simulink model "IPC4M"  (R2015a)
settings: Solver=ode3  SolverMode=SingleTasking  StartTime=0.0  StopTime=30.0  FixedStep=1e-2  RelTol=1e-7
values from neighbouring files (symbols this model uses):
  d = 5    [IPC4Minit.m]
  delta = 5    [IPC4Minit.m]
  g = [0;0;-9.81]    [IPC4Minit.m]
  j0 = 10    [IPC4Minit.m]
  j1 = 10    [IPC4Minit.m]
  j2 = 10    [IPC4Minit.m]
  j3 = 10    [IPC4Minit.m]
  j4 = 10    [IPC4Minit.m]
  k = 10    [IPC4Minit.m]
  kappa = 10    [IPC4Minit.m]
  Kc = 10    [IPC4Minit.m]
  l = [1 1 1 1]    [IPC4Minit.m]
  m0 = 10    [IPC4Minit.m]
  m1 = 10    [IPC4Minit.m]
  m2 = 10    [IPC4Minit.m]
  m3 = 10    [IPC4Minit.m]
  m4 = 10    [IPC4Minit.m]
libraries: aerolibutil x4, dspinverses x3, simulink x1
settings Model: CovSFcnEnable=off  Creator=Martin  LastModifiedBy=mangerer
settings SolverCC: ZeroCrossAlgorithm=Adaptive
settings DataIOCC: LimitDataPoints=off
settings OptimizationCC: BlockReduction=off  BooleanDataType=off
settings DebuggingCC: SaveWithParameterizedLinksMsg=none  UnderspecifiedInitializationDetection=Classic  MergeDetectMultiDrivingBlocksExec=none  SignalResolutionControl=TryResolveAllWithWarning
settings HardwareCC: TargetBitPerLong=64  TargetBitPerPointer=64  TargetLongLongMode=on  TargetIntDivRoundTo=Zero  TargetEndianess=LittleEndian  TargetWordSize=64  TargetHWDeviceType=MATLAB Host  ProdEqTarget=off

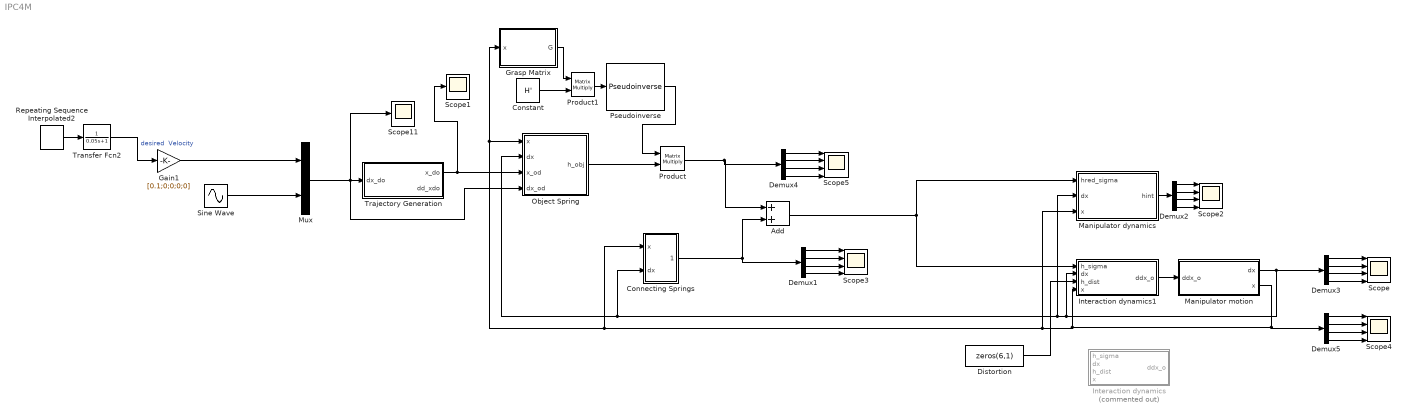
== system IPC4M ==
  Add : Sum
  Connecting Springs : Subsystem
  Constant : Constant  Value=H'
  Demux{1..5} (5 alike) : Demux
  Distortion : Constant  Value=zeros(6,1)
  Gain1 : Gain  Gain=[0.1;0;0;0;0]
  Grasp Matrix : MATLAB Function  TreatAsAtomicUnit=on
  Interaction dynamics : Subsystem  Commented=on
  Interaction dynamics1 : Subsystem
  Manipulator dynamics : Subsystem
  Manipulator motion : Subsystem
  Mux : Mux  Inputs=2
  Object Spring : Subsystem
  Product : Product  Multiplication=Matrix(*)
  Product1 : Product  Multiplication=Matrix(*)
  Pseudoinverse : dspinverses/Pseudoinverse  wanterr=off
  Repeating Sequence Interpolated2 : simulink/Sources/Repeating Sequence Interpolated  OutValues=[0 0 1 1 0 0].'  TimeValues=[0 0.1 1.5 2 2.5 3].'  LookUpMeth=Interpolation-Use End Values  tsamp=0.01  OutMin=[]  OutMax=[]  OutDataTypeStr=double  OutputDataTypeScalingMode=double  OutDataType=fixdt(0,8)  OutScaling=2^-10
  Scope{,2..5} (5 alike) : Scope  NumInputPorts=4
      Scope settings: ShowLegends=on  TimeRange=3  YMin=-15~-12.5~-12.5~-15  YMax=15~15~15~15
      Scope2 settings: ShowLegends=on  TimeRange=10  YMin=-150~-150~-150~-150  YMax=150~150~150~150  SaveName=ScopeData2
      Scope3 settings: ShowLegends=on  TimeRange=3  YMin=-15~-12.5~-12.5~-15  YMax=15~15~15~15  SaveName=ScopeData13
      Scope4 settings: ShowLegends=on  YMin=-5~-5~-5~-5  YMax=5~5~5~5  SaveName=ScopeData10
      Scope5 settings: ShowLegends=on  TimeRange=3  YMin=-15~-12.5~-12.5~-15  YMax=15~15~15~15  SaveName=ScopeData16
  Scope1 : Scope
      settings: YMin=0  YMax=0.9
  Scope11 : Scope
      settings: YMin=0.9984  YMax=1  SaveName=ScopeData26
  Sine Wave : Sin  Amplitude=0  Frequency=1*pi  SampleTime=0
  Trajectory Generation : Subsystem
  Transfer Fcn2 : TransferFcn  Denominator=[0.05 1]
  wires:
  Manipulator dynamics/1(hint) -> Demux2/1
  Demux2/1 -> Scope2/1
  Demux2/2 -> Scope2/2
  Demux2/4 -> Scope2/4
  Demux3/1 -> Scope/1
  Demux3/2 -> Scope/2
  Demux3/3 -> Scope/3
  Demux3/4 -> Scope/4
  Demux5/1 -> Scope4/1
  Demux5/2 -> Scope4/2
  Demux5/3 -> Scope4/3
  Demux5/4 -> Scope4/4
  Gain1/1 -> Mux/1
  Manipulator motion/1(dx) -> Demux3/1, Connecting Springs/2(dx), Object Spring/2(dx), Manipulator dynamics/2(dx), Interaction dynamics1/2(dx)
  Mux/1 -> Scope11/1, Object Spring/4(dx_od), Trajectory Generation/1(dx_do)
  Manipulator motion/2(x) -> Demux5/1, Grasp Matrix/1(x), Object Spring/1(x), Connecting Springs/1(x), Manipulator dynamics/3(x), Interaction dynamics1/4(x)
  Sine Wave/1 -> Mux/2
  Demux2/3 -> Scope2/3
  Interaction dynamics1/1(ddx_o) -> Manipulator motion/1(ddx_o)
  Distortion/1 -> Interaction dynamics1/3(h_dist)
  Trajectory Generation/1(x_do) -> Scope1/1, Object Spring/3(x_od)
  Object Spring/1(h_obj) -> Product/2
  Add/1 -> Manipulator dynamics/1(hred_sigma), Interaction dynamics1/1(h_sigma)
  Repeating Sequence Interpolated2/1 -> Transfer Fcn2/1
  Transfer Fcn2/1 -> Gain1/1  "desired  Velocity"
  Demux1/1 -> Scope3/1
  Demux1/2 -> Scope3/2
  Demux1/3 -> Scope3/3
  Demux1/4 -> Scope3/4
  Connecting Springs/1(h_con) -> Add/2, Demux1/1
  Demux4/1 -> Scope5/1
  Demux4/2 -> Scope5/2
  Demux4/3 -> Scope5/3
  Demux4/4 -> Scope5/4
  Product/1 -> Demux4/1, Add/1
  Grasp Matrix/1(G) -> Product1/1
  Constant/1 -> Product1/2
  Product1/1 -> Pseudoinverse/1
  Pseudoinverse/1 -> Product/1

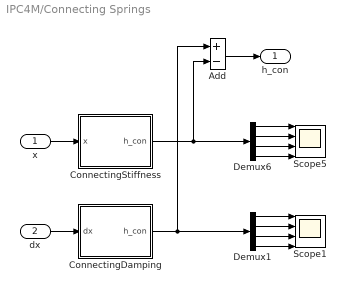
== system IPC4M/Connecting Springs ==
  x : Inport
  dx : Inport  Port=2
  Add : Sum  Inputs=+-
  ConnectingDamping : MATLAB Function  TreatAsAtomicUnit=on
  ConnectingStiffness : MATLAB Function  TreatAsAtomicUnit=on
  Demux1 : Demux
  Demux6 : Demux
  Scope1 : Scope  NumInputPorts=4
      settings: ShowLegends=on  YMin=-10~-50~-80~-80  YMax=80~80~10~50  SaveName=ScopeData12
  Scope5 : Scope  NumInputPorts=4
      settings: ShowLegends=on  YMin=-10~-50~-80~-80  YMax=80~80~10~50  SaveName=ScopeData11
  h_con : Outport
  wires:
  Demux6/1 -> Scope5/1
  Demux6/2 -> Scope5/2
  Demux6/3 -> Scope5/3
  Demux6/4 -> Scope5/4
  ConnectingStiffness/1(h_con) -> Add/2, Demux6/1
  Demux1/1 -> Scope1/1
  Demux1/2 -> Scope1/2
  Demux1/3 -> Scope1/3
  Demux1/4 -> Scope1/4
  ConnectingDamping/1(h_con) -> Add/1, Demux1/1
  x/1 -> ConnectingStiffness/1(x)
  dx/1 -> ConnectingDamping/1(dx)
  Add/1 -> h_con/1

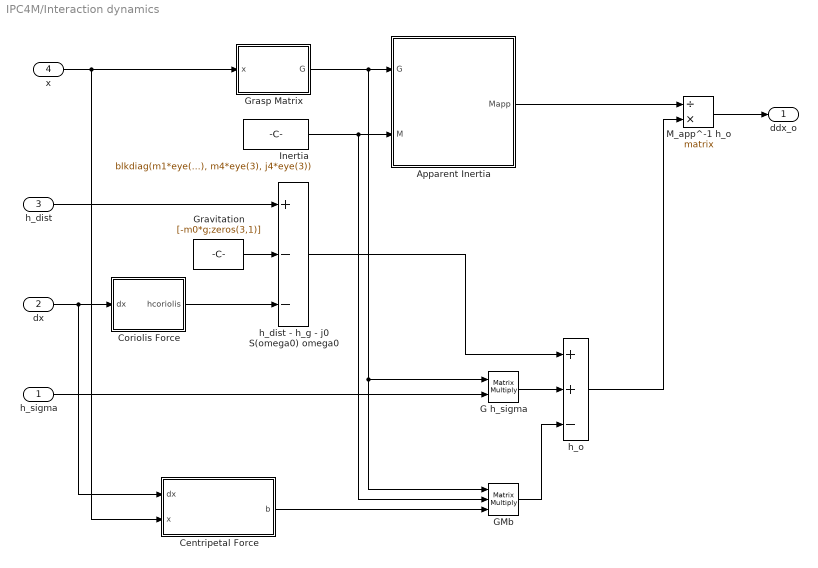
== system IPC4M/Interaction dynamics ==
  h_sigma : Inport
  dx : Inport  Port=2
  h_dist : Inport  Port=3
  x : Inport  Port=4
  Apparent Inertia : MATLAB Function  TreatAsAtomicUnit=on
  Centripetal Force : MATLAB Function  TreatAsAtomicUnit=on
  Coriolis Force : MATLAB Function  TreatAsAtomicUnit=on
  G h_sigma : Product  Multiplication=Matrix(*)
  GMb : Product  Inputs=***  Multiplication=Matrix(*)
  Grasp Matrix : MATLAB Function  TreatAsAtomicUnit=on
  Gravitation : Constant  Value=[-m0*g;zeros(3,1)]
  Inertia : Constant  Value=blkdiag(m1*eye(3), j1*eye(3), m2*eye(3), j2*eye(3), m3*eye(3), j3*eye(3), m4*eye(3), j4*eye(3))
  M_app^-1 h_o : Product  Inputs=/*  Multiplication=Matrix(*)
  "h_dist - h_g - j0 S(omega0) omega0 " : Sum  Inputs=+--
  h_o : Sum  Inputs=++-
  ddx_o : Outport
  wires:
  Grasp Matrix/1(G) -> G h_sigma/1, GMb/1, Apparent Inertia/1(G)
  Inertia/1 -> GMb/2, Apparent Inertia/2(M)
  Apparent Inertia/1(Mapp) -> M_app^-1 h_o/1
  h_o/1 -> M_app^-1 h_o/2
  G h_sigma/1 -> h_o/2
  h_sigma/1 -> G h_sigma/2
  "h_dist - h_g - j0 S(omega0) omega0 "/1 -> h_o/1
  h_dist/1 -> "h_dist - h_g - j0 S(omega0) omega0 "/1
  Gravitation/1 -> "h_dist - h_g - j0 S(omega0) omega0 "/2
  dx/1 -> Centripetal Force/1(dx), Coriolis Force/1(dx)
  Coriolis Force/1(hcoriolis) -> "h_dist - h_g - j0 S(omega0) omega0 "/3
  GMb/1 -> h_o/3
  Centripetal Force/1(b) -> GMb/3
  M_app^-1 h_o/1 -> ddx_o/1
  x/1 -> Centripetal Force/2(x), Grasp Matrix/1(x)

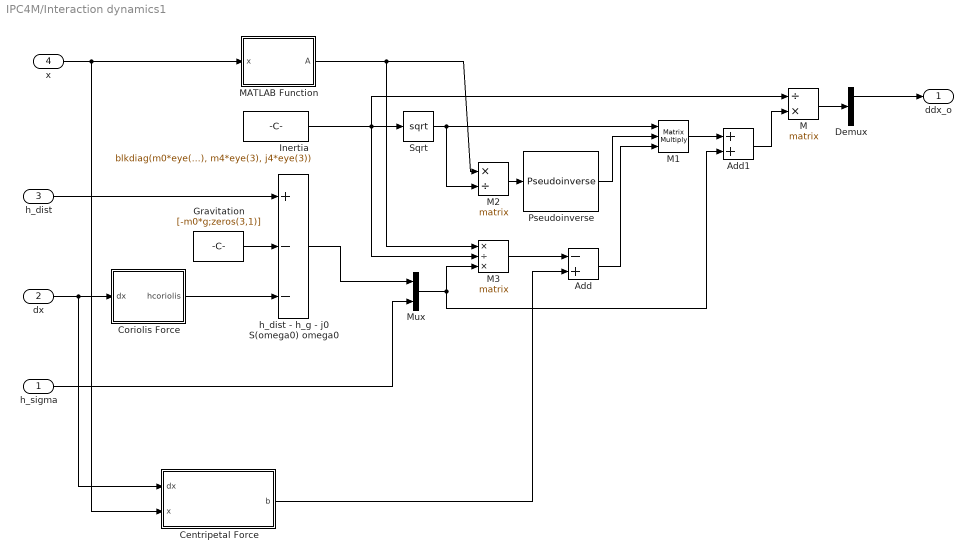
== system IPC4M/Interaction dynamics1 ==
  h_sigma : Inport
  dx : Inport  Port=2
  h_dist : Inport  Port=3
  x : Inport  Port=4
  Add : Sum  Inputs=-+
  Add1 : Sum
  Centripetal Force : MATLAB Function  TreatAsAtomicUnit=on
  Coriolis Force : MATLAB Function  TreatAsAtomicUnit=on
  Demux : Demux  Outputs=5
  Gravitation : Constant  Value=[-m0*g;zeros(3,1)]
  Inertia : Constant  Value=blkdiag(m0*eye(3),j0*eye(3),m1*eye(3), j1*eye(3), m2*eye(3), j2*eye(3), m3*eye(3), j3*eye(3), m4*eye(3), j4*eye(3))
  M : Product  Inputs=/*  Multiplication=Matrix(*)
  M1 : Product  Inputs=***  Multiplication=Matrix(*)
  M2 : Product  Inputs=*/  Multiplication=Matrix(*)
  M3 : Product  Inputs=*/*  Multiplication=Matrix(*)
  MATLAB Function : MATLAB Function  TreatAsAtomicUnit=on
  Mux : Mux  Inputs=2
  Pseudoinverse : dspinverses/Pseudoinverse  wanterr=off
  Sqrt : Sqrt  SaturateOnIntegerOverflow=on
  "h_dist - h_g - j0 S(omega0) omega0 " : Sum  Inputs=+--
  ddx_o : Outport
  wires:
  h_dist/1 -> "h_dist - h_g - j0 S(omega0) omega0 "/1
  Gravitation/1 -> "h_dist - h_g - j0 S(omega0) omega0 "/2
  dx/1 -> Centripetal Force/1(dx), Coriolis Force/1(dx)
  Coriolis Force/1(hcoriolis) -> "h_dist - h_g - j0 S(omega0) omega0 "/3
  x/1 -> MATLAB Function/1(x), Centripetal Force/2(x)
  Inertia/1 -> M/1, M3/2, Sqrt/1
  Sqrt/1 -> M2/2, M1/1
  MATLAB Function/1(A) -> M3/1, M2/1
  M2/1 -> Pseudoinverse/1
  Pseudoinverse/1 -> M1/2
  Add/1 -> M1/3
  Centripetal Force/1(b) -> Add/2
  M3/1 -> Add/1
  Mux/1 -> Add1/2, M3/3
  "h_dist - h_g - j0 S(omega0) omega0 "/1 -> Mux/1
  h_sigma/1 -> Mux/2
  M/1 -> Demux/1
  Demux/1 -> ddx_o/1
  M1/1 -> Add1/1
  Add1/1 -> M/2

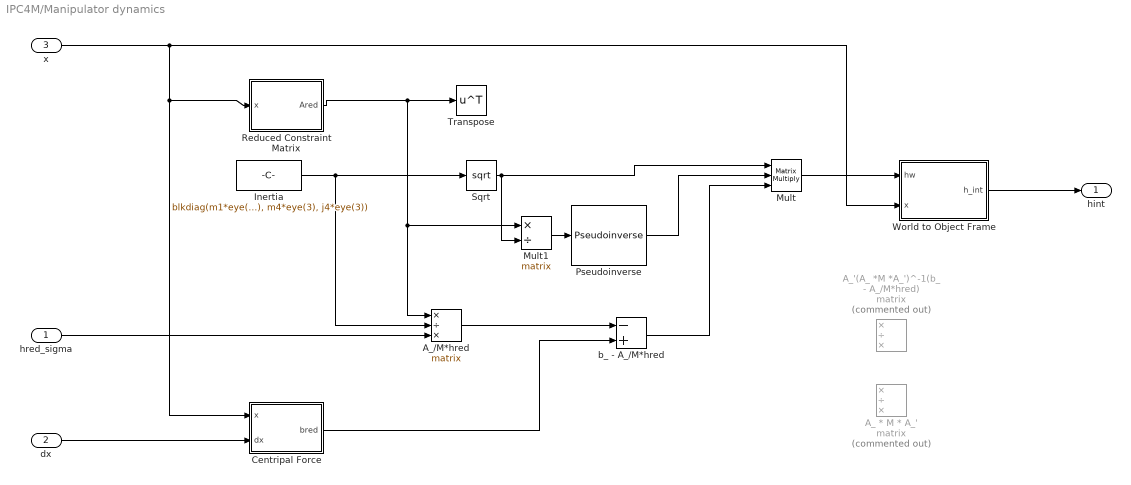
== system IPC4M/Manipulator dynamics ==
  hred_sigma : Inport
  dx : Inport  Port=2
  x : Inport  Port=3
  A_ * M * A_' : Product  Commented=on  Inputs=*/*  Multiplication=Matrix(*)
  A_'(A_ *M *A_')^-1(b_ - A_/M*hred) : Product  Commented=on  Inputs=*/*  Multiplication=Matrix(*)
  A_/M*hred : Product  Inputs=*/*  Multiplication=Matrix(*)
  Centripal Force : MATLAB Function  TreatAsAtomicUnit=on
  Inertia : Constant  Value=blkdiag(m1*eye(3), j1*eye(3), m2*eye(3), j2*eye(3), m3*eye(3), j3*eye(3), m4*eye(3), j4*eye(3))
  Mult : Product  Inputs=***  Multiplication=Matrix(*)
  Mult1 : Product  Inputs=*/  Multiplication=Matrix(*)
  Pseudoinverse : dspinverses/Pseudoinverse  wanterr=off
  Reduced Constraint Matrix : MATLAB Function  TreatAsAtomicUnit=on
  Sqrt : Sqrt  SaturateOnIntegerOverflow=on
  Transpose : Math  Operator=transpose  SaturateOnIntegerOverflow=on
  World to Object Frame : MATLAB Function  TreatAsAtomicUnit=on
  b_ - A_/M*hred : Sum  Inputs=-+
  hint : Outport
  wires:
  Reduced Constraint Matrix/1(Ared) -> Transpose/1, A_/M*hred/1, Mult1/1
  Inertia/1 -> Sqrt/1, A_/M*hred/2
  dx/1 -> Centripal Force/2(dx)
  A_/M*hred/1 -> b_ - A_/M*hred/1
  hred_sigma/1 -> A_/M*hred/3
  World to Object Frame/1(h_int) -> hint/1
  x/1 -> Centripal Force/1(x), Reduced Constraint Matrix/1(x), World to Object Frame/2(x)
  Centripal Force/1(bred) -> b_ - A_/M*hred/2
  Mult/1 -> World to Object Frame/1(hw)
  b_ - A_/M*hred/1 -> Mult/3
  Sqrt/1 -> Mult1/2, Mult/1
  Mult1/1 -> Pseudoinverse/1
  Pseudoinverse/1 -> Mult/2

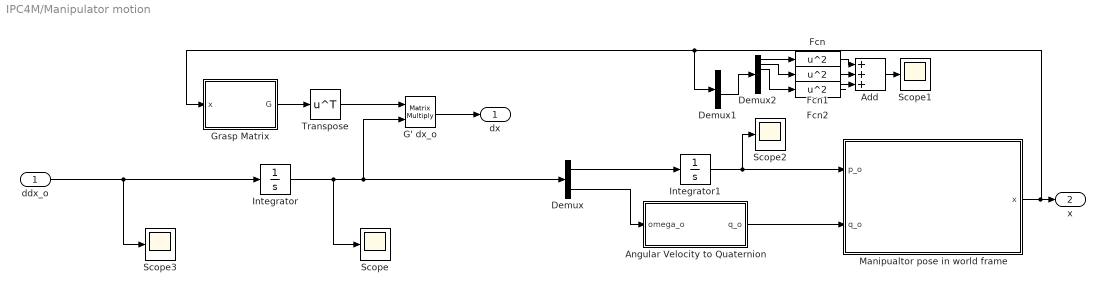
== system IPC4M/Manipulator motion ==
  ddx_o : Inport
  Add : Sum  Inputs=+++
  Angular Velocity to Quaternion : Subsystem
  Demux : Demux  Outputs=2
  Demux1 : Demux
  Demux2 : Demux  Outputs=7
  Fcn : Fcn  Expr=u^2
  Fcn1 : Fcn  Expr=u^2
  Fcn2 : Fcn  Expr=u^2
  G' dx_o : Product  Multiplication=Matrix(*)
  Grasp Matrix : MATLAB Function  TreatAsAtomicUnit=on
  Integrator : Integrator  InitialCondition=zeros(6,1)
  Integrator1 : Integrator  InitialCondition=[0 0 0]'
  Manipualtor pose in world frame : MATLAB Function  TreatAsAtomicUnit=on
  Scope{,1..3} (4 alike) : Scope
      Scope settings: ShowLegends=on  TimeRange=30  YMin=-2.5  YMax=2.5  SaveName=ScopeData14
      Scope1 settings: YMin=0.7  YMax=0.9  SaveName=ScopeData15
      Scope2 settings: YMin=-1  YMax=1  SaveName=ScopeData6
      Scope3 settings: SaveName=ScopeData7
  Transpose : Math  Operator=transpose  SaturateOnIntegerOverflow=on
  dx : Outport
  x : Outport  Port=2
  wires:
  ddx_o/1 -> Scope3/1, Integrator/1
  Integrator/1 -> Scope/1, G' dx_o/2, Demux/1
  Grasp Matrix/1(G) -> Transpose/1
  Transpose/1 -> G' dx_o/1
  G' dx_o/1 -> dx/1
  Demux/2 -> Angular Velocity to Quaternion/1(omega_o)
  Demux/1 -> Integrator1/1
  Integrator1/1 -> Scope2/1, Manipualtor pose in world frame/1(p_o)
  Manipualtor pose in world frame/1(x) -> Demux1/1, Grasp Matrix/1(x), x/1
  Angular Velocity to Quaternion/1(q_o) -> Manipualtor pose in world frame/2(q_o)
  Add/1 -> Scope1/1
  Fcn/1 -> Add/1
  Fcn1/1 -> Add/2
  Fcn2/1 -> Add/3
  Demux2/1 -> Fcn/1
  Demux2/2 -> Fcn1/1
  Demux2/3 -> Fcn2/1
  Demux1/3 -> Demux2/1

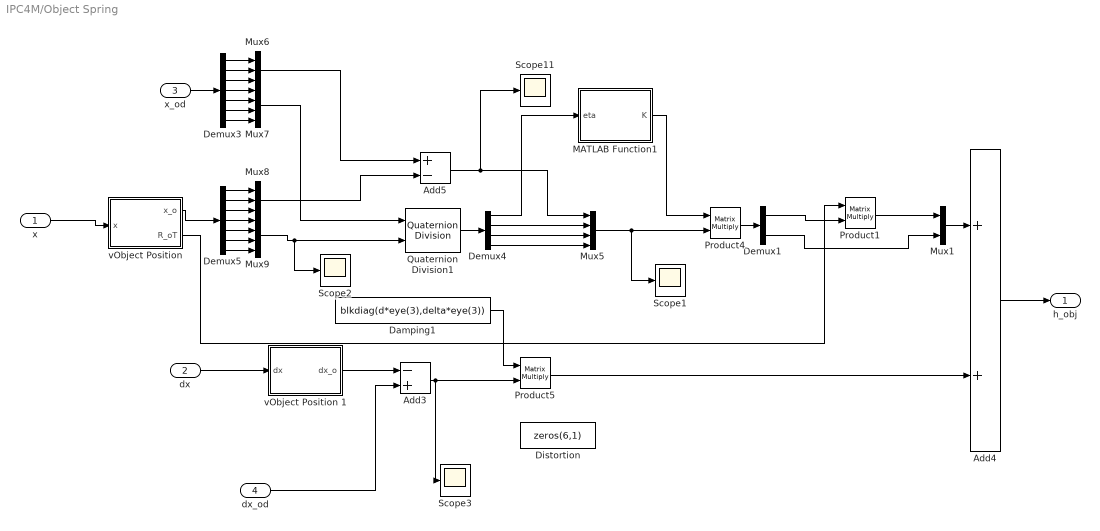
== system IPC4M/Object Spring ==
  x : Inport
  dx : Inport  Port=2
  x_od : Inport  Port=3
  dx_od : Inport  Port=4
  Add3 : Sum  Inputs=-+
  Add4 : Sum
  Add5 : Sum  Inputs=+-
  Damping1 : Constant  Value=blkdiag(d*eye(3),delta*eye(3))
  Demux1 : Demux  Outputs=2
  Demux3 : Demux  Outputs=7
  Demux4 : Demux
  Demux5 : Demux  Outputs=7
  Distortion : Constant  Value=zeros(6,1)
  MATLAB Function1 : MATLAB Function  TreatAsAtomicUnit=on
  Mux1 : Mux  Inputs=2
  Mux5 : Mux
  Mux6 : Mux  Inputs=3
  Mux7 : Mux
  Mux8 : Mux  Inputs=3
  Mux9 : Mux
  Product1 : Product  Multiplication=Matrix(*)
  Product4 : Product  Multiplication=Matrix(*)
  Product5 : Product  Multiplication=Matrix(*)
  Quaternion Division1 : aerolibutil/Quaternion Division
  Scope{1..3,11} (4 alike) : Scope
      Scope1 settings: ShowLegends=on  YMin=0.9984  YMax=1  SaveName=ScopeData4
      Scope11 settings: YMin=0.9984  YMax=1  SaveName=ScopeData3
      Scope2 settings: YMin=0.9984  YMax=1  SaveName=ScopeData5
      Scope3 settings: YMin=0.9984  YMax=1  SaveName=ScopeData8
  "vObject Position " : MATLAB Function  TreatAsAtomicUnit=on
  vObject Position 1 : MATLAB Function  TreatAsAtomicUnit=on
  h_obj : Outport
  wires:
  Add3/1 -> Product5/2, Scope3/1
  Damping1/1 -> Product5/1
  MATLAB Function1/1(K) -> Product4/1
  Demux4/1 -> MATLAB Function1/1(eta)
  Add5/1 -> Scope11/1, Mux5/1
  Demux4/2 -> Mux5/2
  Demux4/3 -> Mux5/3
  Demux4/4 -> Mux5/4
  Demux3/2 -> Mux6/2
  Demux3/1 -> Mux6/1
  Demux3/3 -> Mux6/3
  Demux3/4 -> Mux7/1
  Demux3/5 -> Mux7/2
  Demux3/6 -> Mux7/3
  Demux3/7 -> Mux7/4
  Demux5/2 -> Mux8/2
  Demux5/1 -> Mux8/1
  Demux5/3 -> Mux8/3
  Demux5/4 -> Mux9/1
  Demux5/5 -> Mux9/2
  Demux5/6 -> Mux9/3
  Demux5/7 -> Mux9/4
  Quaternion Division1/1 -> Demux4/1
  Mux5/1 -> Scope1/1, Product4/2
  Add4/1 -> h_obj/1
  Product5/1 -> Add4/2
  x_od/1 -> Demux3/1
  Mux6/1 -> Add5/1
  Mux7/1 -> Quaternion Division1/1
  Mux8/1 -> Add5/2
  Mux9/1 -> Scope2/1, Quaternion Division1/2
  dx_od/1 -> Add3/2
  "vObject Position "/1(x_o) -> Demux5/1
  x/1 -> "vObject Position "/1(x)
  vObject Position 1/1(dx_o) -> Add3/1
  dx/1 -> vObject Position 1/1(dx)
  Mux1/1 -> Add4/1
  Product1/1 -> Mux1/1
  Product4/1 -> Demux1/1
  Demux1/1 -> Product1/2
  Demux1/2 -> Mux1/2
  "vObject Position "/2(R_oT) -> Product1/1

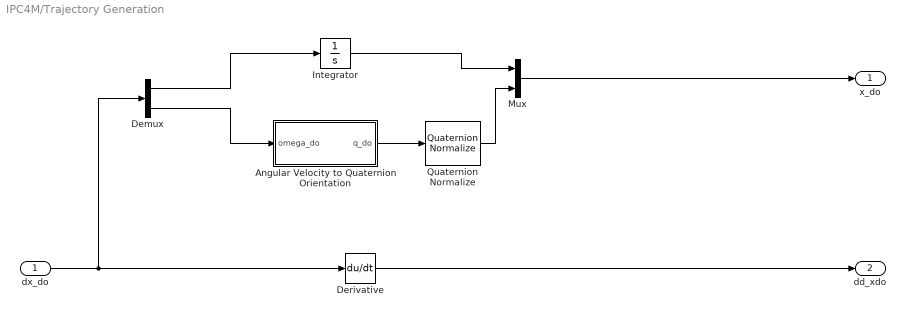
== system IPC4M/Trajectory Generation ==
  dx_do : Inport
  Angular Velocity to Quaternion Orientation : Subsystem
  Demux : Demux  Outputs=2
  Derivative : Derivative
  Integrator : Integrator  InitialCondition=zeros(3,1)
  Mux : Mux  Inputs=2
  Quaternion Normalize : aerolibutil/Quaternion Normalize
  x_do : Outport
  dd_xdo : Outport  Port=2
  wires:
  dx_do/1 -> Derivative/1, Demux/1
  Demux/2 -> Angular Velocity to Quaternion Orientation/1(omega_do)
  Demux/1 -> Integrator/1
  Angular Velocity to Quaternion Orientation/1(q_do) -> Quaternion Normalize/1
  Integrator/1 -> Mux/1
  Mux/1 -> x_do/1
  Derivative/1 -> dd_xdo/1
  Quaternion Normalize/1 -> Mux/2

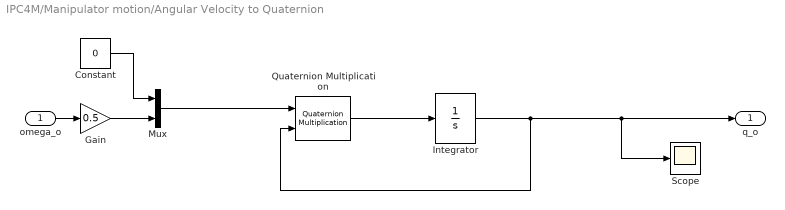
== system IPC4M/Manipulator motion/Angular Velocity to Quaternion ==
  omega_o : Inport
  Constant : Constant  Value=0
  Gain : Gain  Gain=0.5
  Integrator : Integrator  InitialCondition=[1; 0; 0; 0]
  Mux : Mux  Inputs=2
  Quaternion Multiplication : aerolibutil/Quaternion Multiplication
  Scope : Scope
      settings: ShowLegends=on  SaveName=ScopeData9
  q_o : Outport
  wires:
  omega_o/1 -> Gain/1
  Gain/1 -> Mux/2
  Constant/1 -> Mux/1
  Quaternion Multiplication/1 -> Integrator/1
  Integrator/1 -> Quaternion Multiplication/2, q_o/1, Scope/1
  Mux/1 -> Quaternion Multiplication/1

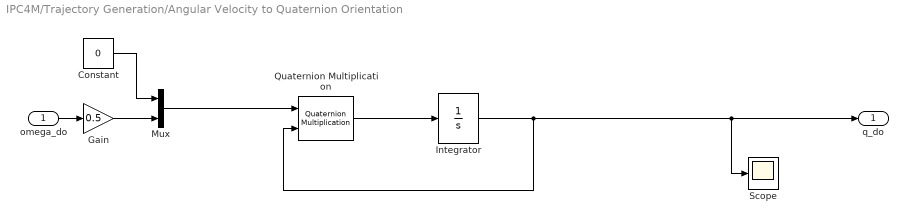
== system IPC4M/Trajectory Generation/Angular Velocity to Quaternion Orientation ==
  omega_do : Inport
  Constant : Constant  Value=0
  Gain : Gain  Gain=0.5
  Integrator : Integrator  InitialCondition=[0.7769; 0; 0; 0.4551]
  Mux : Mux  Inputs=2
  Quaternion Multiplication : aerolibutil/Quaternion Multiplication
  Scope : Scope
      settings: ShowLegends=on  SaveName=ScopeData9
  q_do : Outport
  wires:
  omega_do/1 -> Gain/1
  Gain/1 -> Mux/2
  Constant/1 -> Mux/1
  Quaternion Multiplication/1 -> Integrator/1
  Integrator/1 -> Quaternion Multiplication/2, Scope/1, q_do/1
  Mux/1 -> Quaternion Multiplication/1

== matlab function IPC4M/Object Spring/vObject Position  ==
  data: x_o output; x input; R_oT output
function [x_o,R_oT]= vObjectPose(x)
p1 = x(1:3); p2 = x(8:10); p3 = x(15:17); p4 = x(22:24);
r1n = (p1-p3)/norm(p1-p3) + (p2-p4)/norm(p2-p4);
r1 = r1n/norm(r1n);
r3n = skew_sm(p1-p2)*(p2-p4);
r3 = r3n/norm(r3n);
r2 = skew_sm(r3)*r1;
R_oT = [r1 r2 r3]';
q0 = 0.5*sqrt(r1(1)+r2(2)+r3(3));
q1 = (r2(3)-r3(2))/4/q0;
q2 = (r3(1)-r1(3))/4/q0;
q3 = (r1(2)-r2(1))/4/q0;
x_o = [0.25*[eye(3) zeros(3,4) eye(3) zeros(3,4) eye(3) zeros(3,4) eye(3) zeros(3,4)] * x;
        q0;q1;q2;q3];

== matlab function IPC4M/Object Spring/vObject Position 1 ==
  data: dx_o output; dx input
function dx_o = vObjectVelocity(dx)
dx_o = [0.25*[eye(3) zeros(3) eye(3) zeros(3) eye(3) zeros(3) eye(3) zeros(3)] * dx;
        dx(4:6)];

== matlab function IPC4M/Interaction dynamics1/MATLAB Function ==
  data: r parameter; A output; x input
function A = ConstraintMatrix(r,x)
A = [-eye(3) skew_sm(quatrot(x(4:7),r(1:3))) eye(3) zeros(3,21);
        zeros(3) -eye(3) zeros(3) eye(3) zeros(3,18);
        -eye(3) skew_sm(quatrot(x(4:7),r(4:6))) zeros(3,6) eye(3) zeros(3,15);
        zeros(3) -eye(3) zeros(3,9) eye(3) zeros(3,12);
        -eye(3) skew_sm(quatrot(x(4:7),r(7:9))) zeros(3,12) eye(3) zeros(3,9);
        zeros(3) -eye(3) zeros(3,15) eye(3) zeros(3,6);
        -eye(3) skew_sm(quatrot(x(4:7),r(10:12))) zeros(3,18) eye(3) zeros(3);
        zeros(3) -eye(3) zeros(3,21) eye(3)];

== matlab function IPC4M/Interaction dynamics1/Centripetal Force ==
  data: dx input; b output; r parameter; x input
function b = centripetalforce(dx,r,x)
b = [skew_sm(dx(4:6))*skew_sm(dx(4:6))*quatrot(x(4:7),r(1:3));
     zeros(3,1);
     skew_sm(dx(4:6))*skew_sm(dx(4:6))*quatrot(x(4:7),r(4:6));
     zeros(3,1);
     skew_sm(dx(4:6))*skew_sm(dx(4:6))*quatrot(x(4:7),r(7:9));
     zeros(3,1);
     skew_sm(dx(4:6))*skew_sm(dx(4:6))*quatrot(x(4:7),r(10:12));
     zeros(3,1)];

== matlab function IPC4M/Interaction dynamics1/Coriolis Force ==
  data: dx input; hcoriolis output; j0 parameter; m0 parameter
function hcoriolis = CoriolisForce(dx,j0,m0)
hcoriolis = [m0*skew_sm(dx(4:6))*dx(1:3);
        j0*skew_sm(dx(4:6))*dx(4:6)];

== matlab function IPC4M/Connecting Springs/ConnectingDamping ==
  data: dx input; h_con output; Dc parameter
function h_con = ConnectingDamping(dx,Dc)

H = kron([0.75 -0.25 -0.25 -0.25; -0.25 0.75 -0.25 -0.25; -0.25 -0.25 0.75 -0.25; -0.25 -0.25 -0.25 0.75],eye(3));
v_o = [eye(3) zeros(3) eye(3) zeros(3) eye(3) zeros(3) eye(3) zeros(3)] * dx;
v = [dx(1:3);dx(7:9);dx(13:15);dx(19:21)];
deltav = v - [eye(3);eye(3);eye(3);eye(3)]*v_o;
dmp = Dc*[deltav(1:3);
          deltav(4:6);
          deltav(7:9);
          deltav(10:12)];
f_con = H*dmp;
h_con = [f_con(1:3);zeros(3,1);f_con(4:6);zeros(3,1);f_con(7:9);zeros(3,1);f_con(10:12);zeros(3,1)];

== matlab function IPC4M/Connecting Springs/ConnectingStiffness ==
  data: x input; h_con output; l parameter; Kc parameter
function h_con = ConnectingStiffness(x,l,Kc)

H = kron([0.75 -0.25 -0.25 -0.25; -0.25 0.75 -0.25 -0.25; -0.25 -0.25 0.75 -0.25; -0.25 -0.25 -0.25 0.75],eye(3));
p_o = [eye(3) zeros(3,4) eye(3) zeros(3,4) eye(3) zeros(3,4) eye(3) zeros(3,4)] * x;
p = [x(1:3);x(8:10);x(15:17);x(22:24)];
deltap = p - [eye(3);eye(3);eye(3);eye(3)]*p_o;
stf = Kc*[(norm(deltap(1:3))-l(1))/norm(deltap(1:3))*deltap(1:3);
          (norm(deltap(4:6))-l(2))/norm(deltap(4:6))*deltap(4:6);
          (norm(deltap(7:9))-l(3))/norm(deltap(7:9))*deltap(7:9);
          (norm(deltap(10:12))-l(4))/norm(deltap(10:12))*deltap(10:12)];
f_con = H*stf;
h_con = [f_con(1:3);zeros(3,1);f_con(4:6);zeros(3,1);f_con(7:9);zeros(3,1);f_con(10:12);zeros(3,1)];

== matlab function IPC4M/Grasp Matrix ==
  data: r parameter; G output; x input
function G = GraspMatrix(r,x)
x_o = [eye(3) zeros(3,4) eye(3) zeros(3,4) eye(3) zeros(3,4) eye(3) zeros(3,4)] * x;
G = [eye(3) zeros(3) eye(3) zeros(3) eye(3) zeros(3) eye(3) zeros(3);
    skew_sm(quatrot(x(4:7),x(1:3)-x_o)) eye(3) skew_sm(quatrot(x(4:7),x(8:10)-x_o)) eye(3) skew_sm(quatrot(x(4:7),x(15:17)-x_o)) eye(3) skew_sm(quatrot(x(4:7),x(22:24)-x_o)) eye(3)];

== matlab function IPC4M/Object Spring/MATLAB Function1 ==
  data: eta input; K output; k parameter; kappa parameter
function K = stiffness(eta,k,kappa)
K = blkdiag(k*eye(3),2*eta*kappa*eye(3));

== matlab function IPC4M/Manipulator dynamics/Reduced Constraint Matrix ==
  data: r parameter; Ared output; x input
function Ared = ReducedConstraintMAtrix(r,x)
%x_o = [eye(3) zeros(3,4) eye(3) zeros(3,4) eye(3) zeros(3,4) eye(3) zeros(3,4)] * x;
Ared = [-eye(3) skew_sm(quatrot(x(4:7),r(4:6)-r(1:3))) eye(3) zeros(3,15);
        zeros(3) -eye(3) zeros(3) eye(3) zeros(3,12);
        -eye(3) skew_sm(quatrot(x(4:7),r(7:9)-r(1:3))) zeros(3,6) eye(3) zeros(3,9);
        zeros(3) -eye(3) zeros(3,9) eye(3) zeros(3,6);
        -eye(3) skew_sm(quatrot(x(4:7),r(10:12)-r(1:3))) zeros(3,12) eye(3) zeros(3);
        zeros(3) -eye(3) zeros(3,15) eye(3)];
% Ared = [-eye(3) skew_sm(quatrot(x(4:7),x(8:10)-x(1:3))) eye(3) zeros(3,15);
%         zeros(3) -eye(3) zeros(3) eye(3) zeros(3,12);
%         -eye(3) skew_sm(quatrot(x(4:7),x(15:17)-x(1:3))) zeros(3,6) eye(3) zeros(3,9);
%         zeros(3) -eye(3) zeros(3,9) eye(3) zeros(3,6);
%         -eye(3) skew_sm(quatrot(x(4:7),x(22:24)-x(1:3))) zeros(3,12) eye(3) zeros(3);
%         zeros(3) -eye(3) zeros(3,15) eye(3)];

== matlab function IPC4M/Manipulator dynamics/Centripal Force ==
  data: r parameter; x input; bred output; dx input
function bred = ReducedCentripetalvector(r,x,dx)
bred = [skew_sm(dx(4:6))*skew_sm(dx(4:6))*quatrot(x(4:7),(r(4:6)-r(1:3)));
        zeros(3,1);
        skew_sm(dx(4:6))*skew_sm(dx(4:6))*quatrot(x(4:7),(r(7:9)-r(1:3)));
        zeros(3,1);
        skew_sm(dx(4:6))*skew_sm(dx(4:6))*quatrot(x(4:7),(r(10:12)-r(1:3)));
        zeros(3,1)];
%     bred = [skew_sm(dx(4:6))*skew_sm(dx(4:6))*quatrot(x(4:7),(x(8:10)-x(1:3)));
%         zeros(3,1);
%         skew_sm(dx(4:6))*skew_sm(dx(4:6))*quatrot(x(4:7),(x(15:17)-x(1:3)));
%         zeros(3,1);
%         skew_sm(dx(4:6))*skew_sm(dx(4:6))*quatrot(x(4:7),(x(22:24)-x(1:3)));
%         zeros(3,1)];

== matlab function IPC4M/Interaction dynamics/Apparent Inertia ==
  data: G input; Mapp output; M input; m0 parameter; j0 parameter
function Mapp = ApparentInertia(G,M,m0,j0)
Mapp = blkdiag(m0*eye(3),j0*eye(3)) + G*M*G';

== matlab function IPC4M/Interaction dynamics/Grasp Matrix ==
  data: r parameter; G output; x input
function G = GraspMatrix(r,x)
G = [eye(3) zeros(3) eye(3) zeros(3) eye(3) zeros(3) eye(3) zeros(3);
    skew_sm(quatrot(x(4:7),r(1:3))) eye(3) skew_sm(quatrot(x(4:7),r(4:6))) eye(3) skew_sm(quatrot(x(4:7),r(7:9))) eye(3) skew_sm(quatrot(x(4:7),r(10:12))) eye(3)];

== matlab function IPC4M/Interaction dynamics/Coriolis Force ==
  data: dx input; hcoriolis output; j0 parameter; m0 parameter
function hcoriolis = CoriolisForce(dx,j0,m0)
hcoriolis = [m0*skew_sm(dx(4:6))*dx(1:3);
        j0*skew_sm(dx(4:6))*dx(4:6)];

== matlab function IPC4M/Interaction dynamics/Centripetal Force ==
  data: dx input; b output; r parameter; x input
function b = centripetalforce(dx,r,x)
b = [skew_sm(dx(4:6))*skew_sm(dx(4:6))*quatrot(x(4:7),r(1:3));
     zeros(3,1);
     skew_sm(dx(4:6))*skew_sm(dx(4:6))*quatrot(x(4:7),r(4:6));
     zeros(3,1);
     skew_sm(dx(4:6))*skew_sm(dx(4:6))*quatrot(x(4:7),r(7:9));
     zeros(3,1);
     skew_sm(dx(4:6))*skew_sm(dx(4:6))*quatrot(x(4:7),r(10:12));
     zeros(3,1)];

== matlab function IPC4M/Manipulator motion/Grasp Matrix ==
  data: r parameter; G output; x input
function G = GraspMatrix(r,x)
G = [eye(3) zeros(3) eye(3) zeros(3) eye(3) zeros(3) eye(3) zeros(3);
    skew_sm(quatrot(x(4:7),r(1:3))) eye(3) skew_sm(quatrot(x(4:7),r(4:6))) eye(3) skew_sm(quatrot(x(4:7),r(7:9))) eye(3) skew_sm(quatrot(x(4:7),r(10:12))) eye(3)];

== matlab function IPC4M/Manipulator motion/Manipualtor pose in world frame ==
  data: p_o input; q_o input size=4; x output; r parameter
function x = manipulatorpose(p_o,q_o,r)

x = [p_o + quatrot(q_o,r(1:3));
        q_o;
        p_o + quatrot(q_o,r(4:6));
        q_o;
        p_o + quatrot(q_o,r(7:9));
        q_o;
        p_o + quatrot(q_o,r(10:12));
        q_o ];

== matlab function IPC4M/Manipulator dynamics/World to Object Frame ==
  data: hw input; x input; h_int output
function h_int = inertial2objectFrame(hw,x)

h_int = [quatrot(quatconj(x(4:7)')',hw(1:3));
         hw(4:6);%quatrot(quatconj(x(4:7)')',hw(4:6));
         quatrot(quatconj(x(4:7)')',hw(7:9));
         hw(10:12);%quatrot(quatconj(x(4:7)')',hw(10:12));
         quatrot(quatconj(x(4:7)')',hw(13:15));
         hw(16:18);%quatrot(quatconj(x(4:7)')',hw(16:18));
         quatrot(quatconj(x(4:7)')',hw(19:21));
         hw(22:24)];%quatrot(quatconj(x(4:7)')',hw(22:24));];
